simulink subsystem "KukaVisualizationModel"  (R2021a)
settings: Solver=VariableStepAuto  StartTime=0.0  StopTime=10.0  RelTol=1e-3
libraries: vrlib x1
settings Model: Creator=chiar  LastModifiedBy=chiar

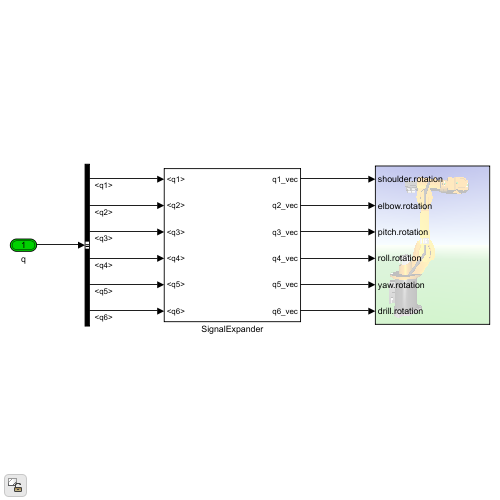
[thumbnail: Simulink's stored preview of the top-level diagram]
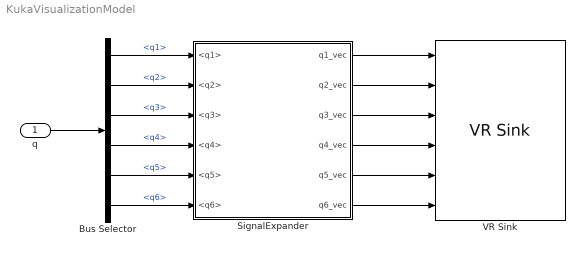
== system KukaVisualizationModel ==
  q : Inport  OutDataTypeStr=Bus: Bus_q
  Bus Selector : BusSelector  OutputSignals=q1,q2,q3,q4,q5,q6
  SignalExpander : Subsystem
  VR Sink : vrlib/VR Sink  InstantiateOnLoad=on  SampleTime=0.1  ViewEnable=on  RemoteChange=off  RemoteView=off  FieldsWritten=shoulder.rotation.4.1.1.double#elbow.rotation.4.1.1.double#pitch.rotation.4.1.1.double#roll.rotation.4.1.1.double#yaw.rotation.4.1.1.double#drill.rotation.4.1.1.double  WorldFileName=D:\cleo\KukaKR6\srcs\wrl\KukaKR6__.WRL  AutoView=off  VideoDimensions=[]  AllowVariableSize=off
  wires:
  q/1 -> Bus Selector/1
  SignalExpander/1(q1_vec) -> VR Sink/1
  SignalExpander/6(q6_vec) -> VR Sink/6
  SignalExpander/5(q5_vec) -> VR Sink/5
  SignalExpander/4(q4_vec) -> VR Sink/4
  SignalExpander/3(q3_vec) -> VR Sink/3
  SignalExpander/2(q2_vec) -> VR Sink/2
  Bus Selector/1 -> SignalExpander/1(<q1>)  "<q1>"
  Bus Selector/2 -> SignalExpander/2(<q2>)  "<q2>"
  Bus Selector/3 -> SignalExpander/3(<q3>)  "<q3>"
  Bus Selector/4 -> SignalExpander/4(<q4>)  "<q4>"
  Bus Selector/5 -> SignalExpander/5(<q5>)  "<q5>"
  Bus Selector/6 -> SignalExpander/6(<q6>)  "<q6>"

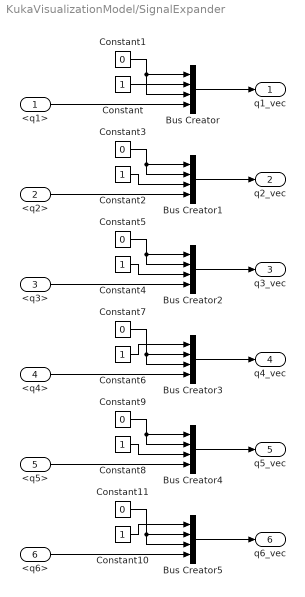
== system KukaVisualizationModel/SignalExpander ==
  <q1> : Inport
  <q2> : Inport  Port=2
  <q3> : Inport  Port=3
  <q4> : Inport  Port=4
  <q5> : Inport  Port=5
  <q6> : Inport  Port=6
  Bus Creator{,1..5} (6 alike) : BusCreator  Inputs=4
  Constant{,2,4,6,8,10} (6 alike) : Constant
  Constant{1,3,5,7,9,11} (6 alike) : Constant  Value=0
  q1_vec : Outport
  q2_vec : Outport  Port=2
  q3_vec : Outport  Port=3
  q4_vec : Outport  Port=4
  q5_vec : Outport  Port=5
  q6_vec : Outport  Port=6
  wires:
  Bus Creator1/1 -> q2_vec/1
  <q6>/1 -> Bus Creator5/4
  Bus Creator3/1 -> q4_vec/1
  <q5>/1 -> Bus Creator4/4
  <q1>/1 -> Bus Creator/4
  Constant/1 -> Bus Creator/2
  <q4>/1 -> Bus Creator3/4
  Bus Creator2/1 -> q3_vec/1
  Constant8/1 -> Bus Creator4/3
  Constant1/1 -> Bus Creator/1, Bus Creator/3
  Constant5/1 -> Bus Creator2/1, Bus Creator2/2
  Constant4/1 -> Bus Creator2/3
  Bus Creator4/1 -> q5_vec/1
  Bus Creator5/1 -> q6_vec/1
  <q2>/1 -> Bus Creator1/4
  Constant9/1 -> Bus Creator4/1, Bus Creator4/2
  Constant10/1 -> Bus Creator5/1
  Bus Creator/1 -> q1_vec/1
  <q3>/1 -> Bus Creator2/4
  Constant6/1 -> Bus Creator3/1
  Constant2/1 -> Bus Creator1/3
  Constant7/1 -> Bus Creator3/2, Bus Creator3/3
  Constant11/1 -> Bus Creator5/2, Bus Creator5/3
  Constant3/1 -> Bus Creator1/1, Bus Creator1/2
